simulink model "model_simple"  (R2022a)
settings: Solver=VariableStepAuto  StartTime=0.0  StopTime=5000  RelTol=1e-3
values from neighbouring files (symbols this model uses):
  drain_area = pi*(drain_d^2)/4    (= 7.85398163397e-05)    [in.m]
  g = 9.8    [in.m]
  pump_speed = 5/6*pump_max_speed    (= 8.33333333333e-05)    [in.m]
  R = -26/16    (= -1.625)    [in.m]
  sonar_height = 0.1    [in.m]
  sonar_signal_time = 20*10^(-6)    (= 2e-05)    [in.m]
  sonar_T = 0.1    [in.m]
  target_area = target_V/target_h    (= 0.025)    [in.m]
  target_h = 0.2    [in.m]
  theta0 = asin(1 - pump_speed/drain_area/sqrt(2*g*target_h))    [in.m]
libraries: slpidlib x1
settings Model: Creator=ilyas  LastModifiedBy=ilyas

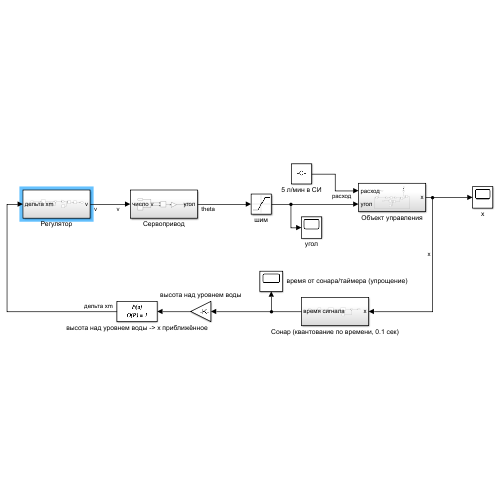
[thumbnail: Simulink's stored preview of the top-level diagram]
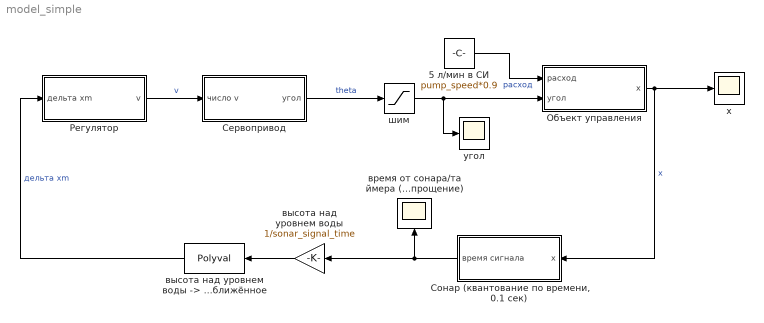
== system model_simple ==
  5 л/мин в СИ : Constant  Value=pump_speed*0.9
  Объект управления : Subsystem
  Регулятор : Subsystem
  Сервопривод : Subsystem
  "Сонар (квантование по времени, 0.1 сек)" : Subsystem
  время от сонара/таймера (упрощение) : Scope
  высота над уровнем воды : Gain  Gain=1/sonar_signal_time
  "высота над уровнем воды -> х приближённое" : Polyval  Coefs=[ -1 (sonar_height)]
  угол : Scope
  х : Scope
  шим : Saturate  UpperLimit=pi  LowerLimit=-pi
  wires:
  Объект управления/1(х) -> "Сонар (квантование по времени, 0.1 сек)"/1(х), х/1  "x"
  "Сонар (квантование по времени, 0.1 сек)"/1(время сигнала) -> высота над уровнем воды/1, время от сонара/таймера (упрощение)/1
  Регулятор/1(v) -> Сервопривод/1(число v)  "v"
  5 л/мин в СИ/1 -> Объект управления/1(расход)  "расход"
  высота над уровнем воды/1 -> "высота над уровнем воды -> х приближённое"/1
  "высота над уровнем воды -> х приближённое"/1 -> Регулятор/1(дельта хm)  "дельта xm"
  шим/1 -> угол/1, Объект управления/2(угол)
  Сервопривод/1(угол) -> шим/1  "theta"

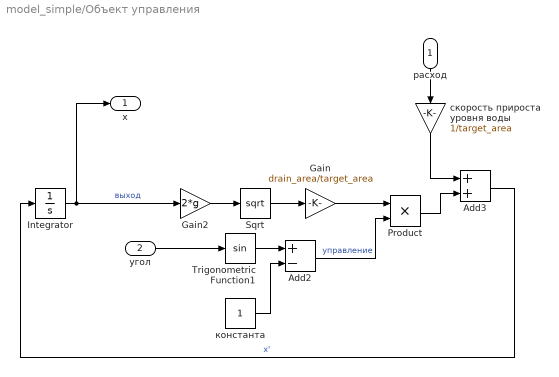
== system model_simple/Объект управления ==
  расход : Inport
  угол : Inport  Port=2
  Add2 : Sum  Inputs=+-
  Add3 : Sum
  Gain : Gain  Gain=drain_area/target_area
  Gain2 : Gain  Gain=2*g
  Integrator : Integrator
  Product : Product
  Sqrt : Sqrt
  Trigonometric Function1 : Trigonometry
  константа : Constant
  скорость прироста уровня воды : Gain  Gain=1/target_area
  х : Outport
  wires:
  скорость прироста уровня воды/1 -> Add3/1
  Gain2/1 -> Sqrt/1
  Add3/1 -> Integrator/1  "x'"
  Add2/1 -> Product/2  "управление"
  Product/1 -> Add3/2
  константа/1 -> Add2/2
  расход/1 -> скорость прироста уровня воды/1
  Integrator/1 -> Gain2/1, х/1  "выход"
  Trigonometric Function1/1 -> Add2/1
  Gain/1 -> Product/1
  Sqrt/1 -> Gain/1
  угол/1 -> Trigonometric Function1/1

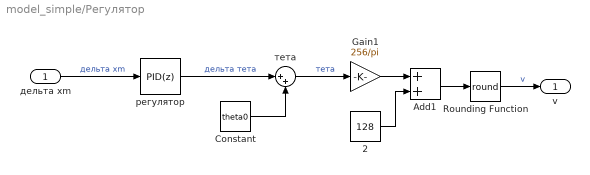
== system model_simple/Регулятор ==
  дельта хm : Inport
  2 : Constant  Value=128
  Add1 : Sum
  Constant : Constant  Value=theta0
  Gain1 : Gain  Gain=256/pi
  Rounding Function : Rounding  Operator=round
  регулятор : slpidlib/PID Controller  Controller=PID  Form=Parallel  TimeDomain=Discrete-time  UseExternalTs=off  SampleTime=-1  IntegratorMethod=Forward Euler  FilterMethod=Forward Euler  ControllerParametersSource=internal  P=R  I=0  UseKiTs=off  D=0  N=100  UseFilter=on  TunerSelectOption=Transfer Function Based (PID Tuner App)  InitialConditionSource=internal  InitialConditionForIntegrator=0  InitialConditionForFilter=0  DifferentiatorICPrevScaledInput=0  ExternalReset=none  TrackingMode=off  Kt=1  LimitOutput=off  SatLimitsSource=internal  UpperSaturationLimit=inf  LowerSaturationLimit=-inf  LinearizeAsGain=off  AntiWindupMode=none  Kb=1  POutMin=[]  POutMax=[]  IOutMin=[]  IOutMax=[]  DOutMin=[]  DOutMax=[]  NOutMin=[]  NOutMax=[]  SumOutMin=[]  SumOutMax=[]  SaturationOutMin=[]  SaturationOutMax=[]  PParamMin=[]  PParamMax=[]  IParamMin=[]  IParamMax=[]  DParamMin=[]  DParamMax=[]  NParamMin=[]  NParamMax=[]  KbParamMin=[]  KbParamMax=[]  KtParamMin=[]  KtParamMax=[]  KbOutMin=[]  KbOutMax=[]  KtOutMin=[]  KtOutMax=[]  IntegratorOutMin=[]  IntegratorOutMax=[]  FilterOutMin=[]  FilterOutMax=[]  SumI1OutMin=[]  SumI1OutMax=[]  SumI2OutMin=[]  SumI2OutMax=[]  SumI3OutMin=[]  SumI3OutMax=[]  SumI4OutMin=[]  SumI4OutMax=[]  SumDOutMin=[]  SumDOutMax=[]  DifferentiatorOutMin=[]  DifferentiatorOutMax=[]  FilterDiffOutCoefMin=[]  FilterDiffOutCoefMax=[]  ReciprocalOutMin=[]  ReciprocalOutMax=[]  SumDenOutMin=[]  SumDenOutMax=[]  SumNumOutMin=[]  SumNumOutMax=[]  DivideOutMin=[]  DivideOutMax=[]  UdiffTsProdOutMin=[]  UdiffTsProdOutMax=[]  NTsProdOutMin=[]  NTsProdOutMax=[]  UintegralTsProdOutMin=[]  UintegralTsProdOutMax=[]  UngainTsProdOutMin=[]  UngainTsProdOutMax=[]  IntegratorContinuousStateAttributes=''  IntegratorStateMustResolveToSignalObject=off  IntegratorRTWStateStorageClass=Auto  FilterContinuousStateAttributes=''  FilterStateMustResolveToSignalObject=off  FilterRTWStateStorageClass=Auto  ParallelPVariant=InternalParameters  IdealPVariant=Disabled  IVariant=InternalParameters  DVariant=InternalParameters  IntegratorVariant=Discrete  SatVariant=Disabled  AWVariant=Passthrough  PCopyVariant=Disabled  TRVariant=Disabled  FdbkBlocksVariant=Forward  IdealPFdbkVariant=Disabled  SatFdbkVariant=Disabled  DerivativeFilterVariant=ForwardEulerFilter  NVariant=InternalParameters  NCopyVariant=Disabled  FilterICVariant=InternalICsFilter  IntegratorICVariant=InternalICs  ExternalResetVariant=Disabled  TRSumVariant=Passthrough  SumFdbkVariant=Disabled  SumVariant=Sum_PID  TsampFilterVariant=InternalTs  TsampNgainVariant=Passthrough  TsampIntegralVariant=Passthrough  ExternalSaturationOutDataTypeStr=Inherit: Same as second input  aMode=0
  тета : Sum  Inputs=|++
  v : Outport
  wires:
  тета/1 -> Gain1/1  "тета"
  Constant/1 -> тета/2
  Gain1/1 -> Add1/1
  2/1 -> Add1/2
  регулятор/1 -> тета/1  "дельта тета"
  дельта хm/1 -> регулятор/1  "дельта xm"
  Add1/1 -> Rounding Function/1
  Rounding Function/1 -> v/1  "v"

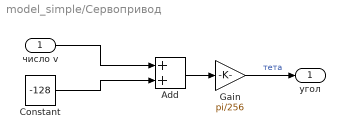
== system model_simple/Сервопривод ==
  число v : Inport
  Add : Sum
  Constant : Constant  Value=-128
  Gain : Gain  Gain=pi/256
  угол : Outport
  wires:
  Constant/1 -> Add/2
  Add/1 -> Gain/1
  число v/1 -> Add/1
  Gain/1 -> угол/1  "тета"

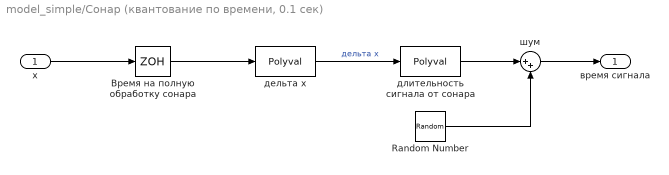
== system model_simple/Сонар (квантование по времени, 0.1 сек) ==
  х : Inport
  Random Number : RandomNumber  Variance=0.0001*sonar_signal_time^2  Seed=10  SampleTime=0.1
  Время на полную обработку сонара : ZeroOrderHold  SampleTime=sonar_T
  дельта х : Polyval  Coefs="[ 1  -target_h]"
  длительность сигнала от сонара : Polyval  Coefs="[ (-1*sonar_signal_time),  (sonar_height*sonar_signal_time)]"
  шум : Sum  Inputs=|++
  время сигнала : Outport
  wires:
  длительность сигнала от сонара/1 -> шум/1
  шум/1 -> время сигнала/1
  Random Number/1 -> шум/2
  х/1 -> Время на полную обработку сонара/1
  Время на полную обработку сонара/1 -> дельта х/1
  дельта х/1 -> длительность сигнала от сонара/1  "дельта x"
